simulink model "NeuroControlExamen"  (R2023b)
settings: Solver=VariableStepAuto  StartTime=0.0  StopTime=10.0  RelTol=1e-3
(part 1 of 3)
settings Model: Creator=rhfue  LastModifiedBy=daroc

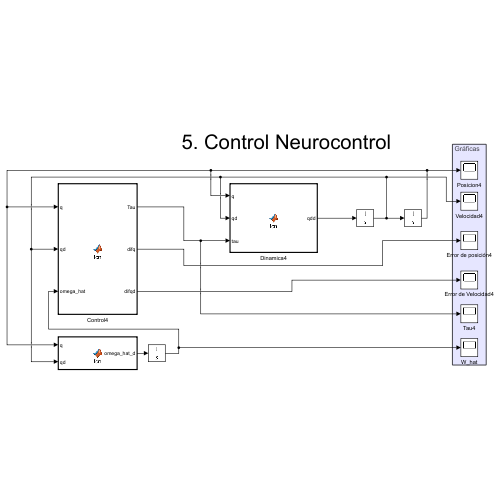
[thumbnail: Simulink's stored preview of the top-level diagram]
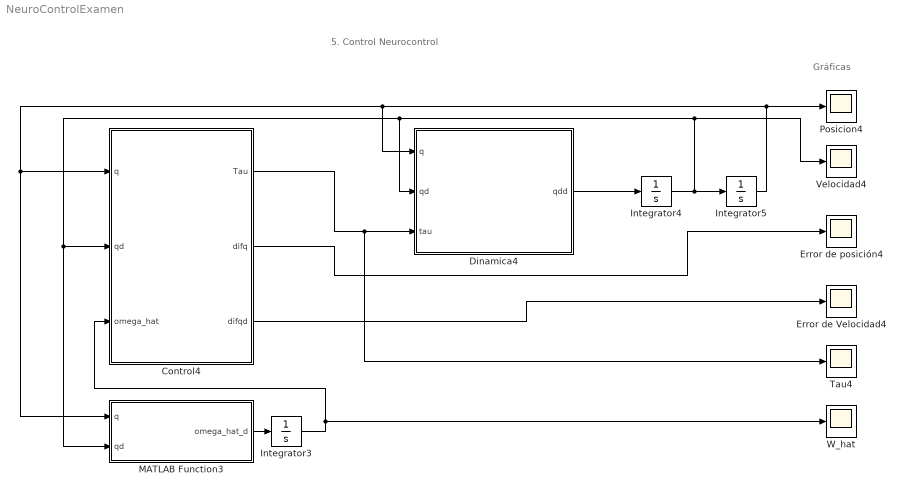
== system NeuroControlExamen ==
  note: 5. Control Neurocontrol
  note: Gráficas
  Control4 : MATLAB Function  TreatAsAtomicUnit=on
  Dinamica4 : MATLAB Function  TreatAsAtomicUnit=on
  Error de Velocidad4 : Scope
  Error de posición4 : Scope
  Integrator3 : Integrator
  Integrator4 : Integrator  InitialCondition=[0;0;0]
  Integrator5 : Integrator  InitialCondition=[0;0;0]
  MATLAB Function3 : MATLAB Function  TreatAsAtomicUnit=on
  Posicion4 : Scope
  Tau4 : Scope
  Velocidad4 : Scope
  W_hat : Scope
  wires:
  Control4/1(Tau) -> Tau4/1, Dinamica4/3(tau)
  MATLAB Function3/1(omega_hat_d) -> Integrator3/1
  Integrator3/1 -> W_hat/1, Control4/3(omega_hat)
  Dinamica4/1(qdd) -> Integrator4/1
  Integrator4/1 -> Integrator5/1, MATLAB Function3/2(qd), Control4/2(qd), Dinamica4/2(qd), Velocidad4/1
  Integrator5/1 -> Posicion4/1, Dinamica4/1(q), Control4/1(q), MATLAB Function3/1(q)
  Control4/2(difq) -> Error de posición4/1
  Control4/3(difqd) -> Error de Velocidad4/1

== matlab function NeuroControlExamen/Control4 ==
  data: q input; Tau output; qd input; difq output; difqd output; omega_hat input
function [Tau, difq, difqd] = fcn(q,qd,omega_hat)

kd=diag([15 15 15]);

alpha = diag([5 5 5]);

q_deseada = [0.3;0.4;0.5];
qd_deseada = [0;0;0];
difq = q-q_deseada;
difqd = qd-qd_deseada;

S = difqd+alpha*difq;

phi = [difq; difqd; q_deseada; qd_deseada; S];

Tau = -kd*S+omega_hat.'*phi;
